simulink model "fofbsim_model"  (Simulink 7.3)
settings: Solver=ode45  StartTime=0.0  StopTime=config_fofbsim.sim_time  MaxStep=config_fofbsim.sim_max_step  RelTol=1e-3
undefined symbols (not defined in the file or in its folder): config_fofbsim, ss_matrices_fofbsim
settings Model: Creator=daniel.tavares  LastModifiedBy=daniel.tavares

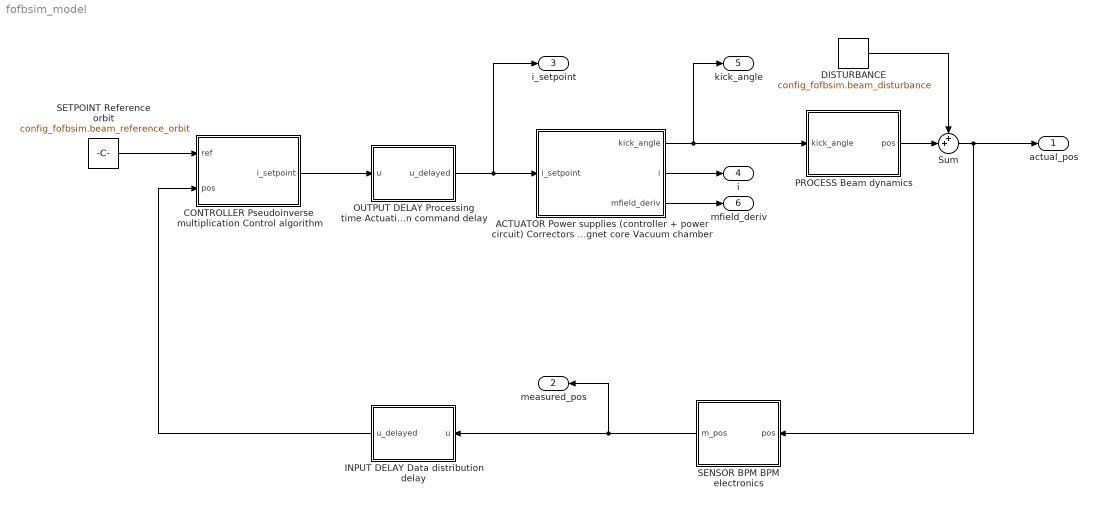
== system fofbsim_model ==
  ACTUATOR Power supplies (controller + power circuit) Correctors Magnet core Vacuum chamber : Subsystem
  CONTROLLER Pseudoinverse multiplication Control algorithm : Subsystem
  DISTURBANCE : FromWorkspace  VariableName=config_fofbsim.beam_disturbance  SampleTime=0  OutputAfterFinalValue=Holding final value
  INPUT DELAY Data distribution delay : Subsystem
  OUTPUT DELAY Processing time Actuation command delay : Subsystem
  PROCESS Beam dynamics : Subsystem
  SENSOR BPM BPM electronics : Subsystem
  SETPOINT Reference orbit : Constant  Value=config_fofbsim.beam_reference_orbit  OutDataType=fixdt(1, 16)  OutScaling=2^0
  Sum : Sum  Inputs=++|  OutDataType=fixdt(1, 16)  OutScaling=2^0
  actual_pos : Outport  OutDataType=fixdt(1, 16)  OutScaling=2^0
  measured_pos : Outport  Port=2  OutDataType=fixdt(1, 16)  OutScaling=2^0
  i_setpoint : Outport  Port=3  OutDataType=fixdt(1, 16)  OutScaling=2^0
  i : Outport  Port=4  OutDataType=fixdt(1, 16)  OutScaling=2^0
  kick_angle : Outport  Port=5  OutDataType=fixdt(1, 16)  OutScaling=2^0
  mfield_deriv : Outport  Port=6
  wires:
  CONTROLLER Pseudoinverse multiplication Control algorithm/1(i_setpoint) -> OUTPUT DELAY Processing time Actuation command delay/1(u)
  SETPOINT Reference orbit/1 -> CONTROLLER Pseudoinverse multiplication Control algorithm/1(ref)
  Sum/1 -> SENSOR BPM BPM electronics/1(pos), actual_pos/1
  PROCESS Beam dynamics/1(pos) -> Sum/2
  ACTUATOR Power supplies (controller + power circuit) Correctors Magnet core Vacuum chamber/1(kick_angle) -> PROCESS Beam dynamics/1(kick_angle), kick_angle/1
  SENSOR BPM BPM electronics/1(m_pos) -> INPUT DELAY Data distribution delay/1(u), measured_pos/1
  INPUT DELAY Data distribution delay/1(u_delayed) -> CONTROLLER Pseudoinverse multiplication Control algorithm/2(pos)
  OUTPUT DELAY Processing time Actuation command delay/1(u_delayed) -> ACTUATOR Power supplies (controller + power circuit) Correctors Magnet core Vacuum chamber/1(i_setpoint), i_setpoint/1
  DISTURBANCE/1 -> Sum/1
  ACTUATOR Power supplies (controller + power circuit) Correctors Magnet core Vacuum chamber/2(i) -> i/1
  ACTUATOR Power supplies (controller + power circuit) Correctors Magnet core Vacuum chamber/3(mfield_deriv) -> mfield_deriv/1

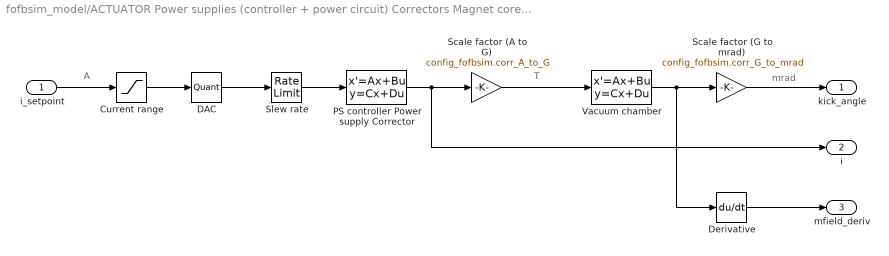
== system fofbsim_model/ACTUATOR Power supplies (controller + power circuit) Correctors Magnet core Vacuum chamber ==
  note: mrad
  note: T
  note: A
  i_setpoint : Inport
  Current range : Saturate  UpperLimit=config_fofbsim.ps_max_current  LowerLimit=config_fofbsim.ps_min_current  OutDataType=fixdt(1, 16)  OutScaling=2^0
  DAC : Quantizer  QuantizationInterval=(config_fofbsim.ps_max_current-config_fofbsim.ps_min_current)/(2^config_fofbsim.ps_dac_bits)  SampleTime=1/config_fofbsim.ps_update_rate
  Derivative : Derivative
  PS controller Power supply Corrector : StateSpace  A=ss_matrices_fofbsim.ps_dynamics.A  B=ss_matrices_fofbsim.ps_dynamics.B  C=ss_matrices_fofbsim.ps_dynamics.C  D=ss_matrices_fofbsim.ps_dynamics.D
  Scale factor (A to G) : Gain  Gain=config_fofbsim.corr_A_to_G  ParameterDataType=fixdt(1, 16)  ParameterScaling=2^0  OutDataType=fixdt(1, 16)  OutScaling=2^0
  Scale factor (G to mrad) : Gain  Gain=config_fofbsim.corr_G_to_mrad  ParameterDataType=fixdt(1, 16)  ParameterScaling=2^0  OutDataType=fixdt(1, 16)  OutScaling=2^0
  Slew rate : RateLimiter  RisingSlewLimit=config_fofbsim.ps_max_slew_rate  FallingSlewLimit=-config_fofbsim.ps_max_slew_rate  SampleTimeMode=inherited
  Vacuum chamber : StateSpace  A=ss_matrices_fofbsim.vac_dynamics.A  B=ss_matrices_fofbsim.vac_dynamics.B  C=ss_matrices_fofbsim.vac_dynamics.C  D=ss_matrices_fofbsim.vac_dynamics.D
  kick_angle : Outport
  i : Outport  Port=2
  mfield_deriv : Outport  Port=3
  wires:
  Vacuum chamber/1 -> Scale factor (G to mrad)/1, Derivative/1
  Current range/1 -> DAC/1
  Scale factor (A to G)/1 -> Vacuum chamber/1
  Derivative/1 -> mfield_deriv/1
  PS controller Power supply Corrector/1 -> i/1, Scale factor (A to G)/1
  DAC/1 -> Slew rate/1
  i_setpoint/1 -> Current range/1
  Slew rate/1 -> PS controller Power supply Corrector/1
  Scale factor (G to mrad)/1 -> kick_angle/1

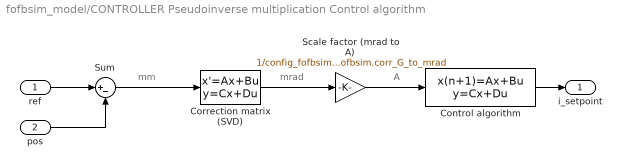
== system fofbsim_model/CONTROLLER Pseudoinverse multiplication Control algorithm ==
  note: mm
  note: A
  note: mrad
  ref : Inport
  pos : Inport  Port=2
  Control algorithm : DiscreteStateSpace  A=ss_matrices_fofbsim.ctrl_algorithm.A  B=ss_matrices_fofbsim.ctrl_algorithm.B  C=ss_matrices_fofbsim.ctrl_algorithm.C  D=ss_matrices_fofbsim.ctrl_algorithm.D  SampleTime=1/config_fofbsim.ps_update_rate
  Correction matrix (SVD) : StateSpace  A=[]  B=[]  C=[]  D=config_fofbsim.ctrl_correction_matrix
  Scale factor (mrad to A) : Gain  Gain=1/config_fofbsim.corr_A_to_G/config_fofbsim.corr_G_to_mrad  ParameterDataType=fixdt(1, 16)  ParameterScaling=2^0  OutDataType=fixdt(1, 16)  OutScaling=2^0
  Sum : Sum  Inputs=|+-  OutDataType=fixdt(1, 16)  OutScaling=2^0
  i_setpoint : Outport
  wires:
  ref/1 -> Sum/1
  pos/1 -> Sum/2
  Correction matrix (SVD)/1 -> Scale factor (mrad to A)/1
  Sum/1 -> Correction matrix (SVD)/1
  Scale factor (mrad to A)/1 -> Control algorithm/1
  Control algorithm/1 -> i_setpoint/1

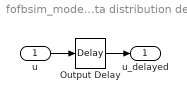
== system fofbsim_model/INPUT DELAY Data distribution delay ==
  u : Inport
  Output Delay : TransportDelay  DelayTime=config_fofbsim.delay_measurement
  u_delayed : Outport
  wires:
  Output Delay/1 -> u_delayed/1
  u/1 -> Output Delay/1

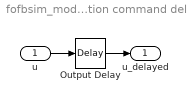
== system fofbsim_model/OUTPUT DELAY Processing time Actuation command delay ==
  u : Inport
  Output Delay : TransportDelay  DelayTime=config_fofbsim.delay_processing + config_fofbsim.delay_actuation
  u_delayed : Outport
  wires:
  u/1 -> Output Delay/1
  Output Delay/1 -> u_delayed/1

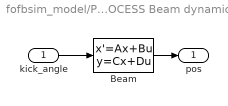
== system fofbsim_model/PROCESS Beam dynamics ==
  kick_angle : Inport
  Beam : StateSpace  A=[]  B=[]  C=[]  D=config_fofbsim.beam_response_matrix
  pos : Outport
  wires:
  kick_angle/1 -> Beam/1
  Beam/1 -> pos/1

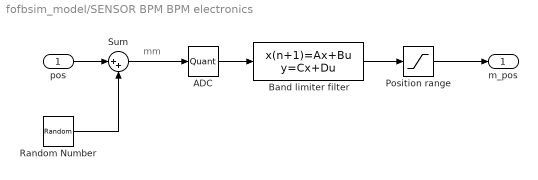
== system fofbsim_model/SENSOR BPM BPM electronics ==
  note: mm
  pos : Inport
  ADC : Quantizer  QuantizationInterval=(config_fofbsim.bpm_max_pos-config_fofbsim.bpm_min_pos)/(2^config_fofbsim.bpm_adc_bits)  SampleTime=1/config_fofbsim.bpm_sampling_rate
  Band limiter filter : DiscreteStateSpace  A=ss_matrices_fofbsim.bpm_filter.A  B=ss_matrices_fofbsim.bpm_filter.B  C=ss_matrices_fofbsim.bpm_filter.C  D=ss_matrices_fofbsim.bpm_filter.D  SampleTime=-1
  Position range : Saturate  UpperLimit=config_fofbsim.bpm_max_pos  LowerLimit=config_fofbsim.bpm_min_pos  OutDataType=fixdt(1, 16)  OutScaling=2^0
  Random Number : RandomNumber  Mean=zeros(size(config_fofbsim.beam_response_matrix,1),1)  Variance=repmat(config_fofbsim.bpm_noise^2,size(config_fofbsim.beam_response_matrix,1),1)  Seed=floor(rand(size(config_fofbsim.beam_response_matrix,1),1)*10000)  SampleTime=1/config_fofbsim.bpm_sampling_rate
  Sum : Sum  Inputs=|++  OutDataType=fixdt(1, 16)  OutScaling=2^0
  m_pos : Outport
  wires:
  pos/1 -> Sum/1
  Sum/1 -> ADC/1
  Random Number/1 -> Sum/2
  Position range/1 -> m_pos/1
  Band limiter filter/1 -> Position range/1
  ADC/1 -> Band limiter filter/1
